simulink model "LaunchSim"  (R2022a)
settings: Solver=VariableStepAuto  StartTime=0.0  StopTime=inf  RelTol=1e-3
values from neighbouring files (symbols this model uses):
  EMFCoefCim = 18.803/1000    (= 0.018803)    [Climbing.m]    (also in Launch.m; Launching.m)
  InputLaunch = 1    [Launch.m]
  loadInertiaLaunch = 6.12 / (2*12.75) + (1.27*0.6*(0.0254^2))/2    (= 0.24024580596)    [Launch.m]
  mechDampingConstantLaunch = (TorqueCoefCim * EMFCoefCim) / TerminalResistanceCim    (= 0.000117850936333)    [Launch.m]
  ResistorTF = 12/(2*pi*1)    (= 1.9098593171)    [Launch.m]    (also in Launching.m = 0.795774715459)
  TerminalInductanceCim = 122/1000000    (= 0.000122)    [Climbing.m]    (also in Launch.m; Launching.m)
  TerminalResistanceCim = 3    [Climbing.m]    (also in Launch.m; Launching.m)
  TorqueCoefCim = 18.803/1000    (= 0.018803)    [Climbing.m]    (also in Launch.m; Launching.m)
  TorqueDisturbanceLaunch = 0    [Launch.m]
libraries: simulink_extras x3, slpidlib x1
settings Model: PacingRate=0.790000  Creator=JD Herlehy  LastModifiedBy=JD Herlehy

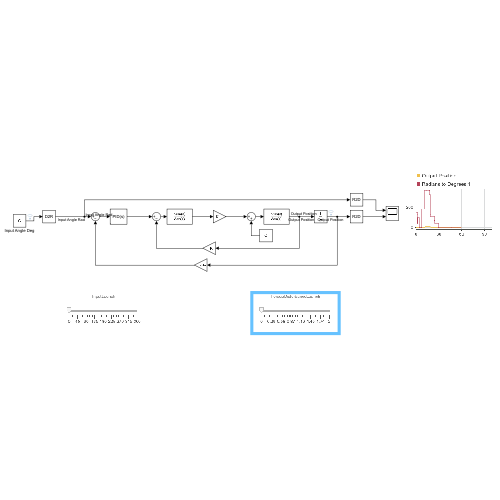
[thumbnail: Simulink's stored preview of the top-level diagram]
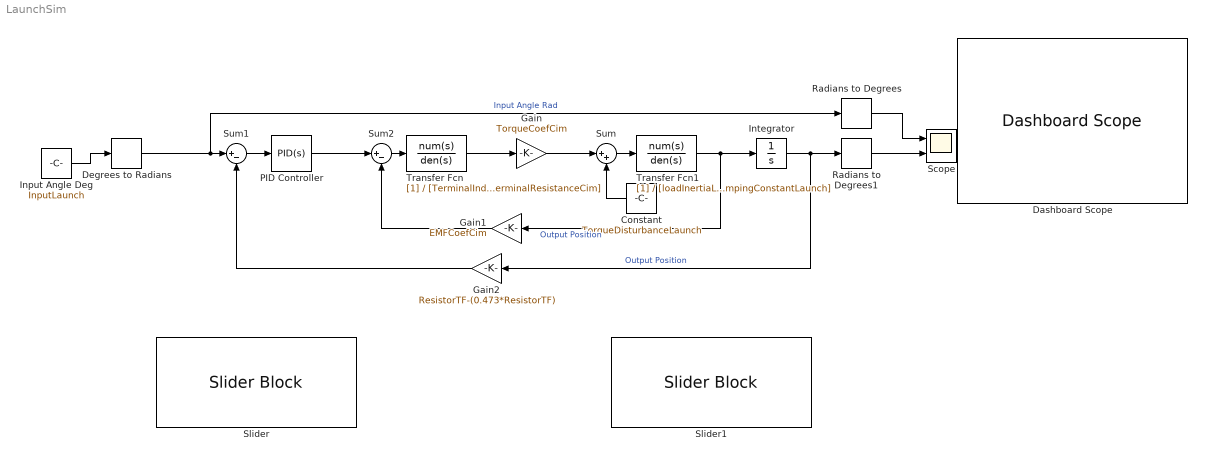
== system LaunchSim ==
  Constant : Constant  Value=TorqueDisturbanceLaunch
  Dashboard Scope : DashboardScope  Ymin=-5  Ymax=420
  Degrees to Radians : simulink_extras/Transformations/Degrees to Radians
  Gain : Gain  Gain=TorqueCoefCim
  Gain1 : Gain  Gain=EMFCoefCim
  Gain2 : Gain  Gain=ResistorTF-(0.473*ResistorTF)
  Input Angle Deg : Constant  Value=InputLaunch
  Integrator : Integrator
  PID Controller : slpidlib/PID Controller  Controller=PID  Form=Parallel  TimeDomain=Continuous-time  UseExternalTs=off  SampleTime=-1  IntegratorMethod=Forward Euler  FilterMethod=Forward Euler  ControllerParametersSource=internal  P=2.03993218165594  I=0.0170011704187148  UseKiTs=off  D=54.3843083130647  N=163.261139434515  UseFilter=on  TunerSelectOption=Transfer Function Based (PID Tuner App)  InitialConditionSource=internal  InitialConditionForIntegrator=0  InitialConditionForFilter=0  DifferentiatorICPrevScaledInput=0  ExternalReset=none  TrackingMode=off  Kt=1  LimitOutput=off  SatLimitsSource=internal  UpperSaturationLimit=inf  LowerSaturationLimit=-inf  LinearizeAsGain=on  AntiWindupMode=none  Kb=1  POutMin=[]  POutMax=[]  IOutMin=[]  IOutMax=[]  DOutMin=[]  DOutMax=[]  NOutMin=[]  NOutMax=[]  SumOutMin=[]  SumOutMax=[]  SaturationOutMin=[]  SaturationOutMax=[]  PParamMin=[]  PParamMax=[]  IParamMin=[]  IParamMax=[]  DParamMin=[]  DParamMax=[]  NParamMin=[]  NParamMax=[]  KbParamMin=[]  KbParamMax=[]  KtParamMin=[]  KtParamMax=[]  KbOutMin=[]  KbOutMax=[]  KtOutMin=[]  KtOutMax=[]  IntegratorOutMin=[]  IntegratorOutMax=[]  FilterOutMin=[]  FilterOutMax=[]  SumI1OutMin=[]  SumI1OutMax=[]  SumI2OutMin=[]  SumI2OutMax=[]  SumI3OutMin=[]  SumI3OutMax=[]  SumI4OutMin=[]  SumI4OutMax=[]  SumDOutMin=[]  SumDOutMax=[]  DifferentiatorOutMin=[]  DifferentiatorOutMax=[]  FilterDiffOutCoefMin=[]  FilterDiffOutCoefMax=[]  ReciprocalOutMin=[]  ReciprocalOutMax=[]  SumDenOutMin=[]  SumDenOutMax=[]  SumNumOutMin=[]  SumNumOutMax=[]  DivideOutMin=[]  DivideOutMax=[]  UdiffTsProdOutMin=[]  UdiffTsProdOutMax=[]  NTsProdOutMin=[]  NTsProdOutMax=[]  UintegralTsProdOutMin=[]  UintegralTsProdOutMax=[]  UngainTsProdOutMin=[]  UngainTsProdOutMax=[]  IntegratorContinuousStateAttributes=''  IntegratorStateMustResolveToSignalObject=off  IntegratorRTWStateStorageClass=Auto  FilterContinuousStateAttributes=''  FilterStateMustResolveToSignalObject=off  FilterRTWStateStorageClass=Auto  ParallelPVariant=InternalParameters  IdealPVariant=Disabled  IVariant=InternalParameters  DVariant=InternalParameters  IntegratorVariant=Continuous  SatVariant=Disabled  AWVariant=Passthrough  PCopyVariant=Disabled  TRVariant=Disabled  FdbkBlocksVariant=Forward  IdealPFdbkVariant=Disabled  SatFdbkVariant=Disabled  DerivativeFilterVariant=ContFilter  NVariant=InternalParameters  NCopyVariant=Disabled  FilterICVariant=InternalICsFilter  IntegratorICVariant=InternalICs  ExternalResetVariant=Disabled  TRSumVariant=Passthrough  SumFdbkVariant=Disabled  SumVariant=Sum_PID  TsampFilterVariant=InternalTs  TsampNgainVariant=Passthrough  TsampIntegralVariant=Passthrough  ExternalSaturationOutDataTypeStr=Inherit: Same as second input  aMode=0
  Radians to Degrees : simulink_extras/Transformations/Radians to Degrees
  Radians to Degrees1 : simulink_extras/Transformations/Radians to Degrees
  Scope : Scope  NumInputPorts=2
  Slider : SliderBlock  ScaleMax=360
  Slider1 : SliderBlock  ScaleMax=2
  Sum : Sum  Inputs=|++
  Sum1 : Sum  Inputs=|+-
  Sum2 : Sum  Inputs=|+-
  Transfer Fcn : TransferFcn  Denominator=[TerminalInductanceCim TerminalResistanceCim]
  Transfer Fcn1 : TransferFcn  Denominator=[loadInertiaLaunch mechDampingConstantLaunch]
  wires:
  Transfer Fcn/1 -> Gain/1
  Gain/1 -> Sum/1
  Sum/1 -> Transfer Fcn1/1
  Input Angle Deg/1 -> Degrees to Radians/1
  Constant/1 -> Sum/2
  Gain1/1 -> Sum2/2
  Sum2/1 -> Transfer Fcn/1
  Gain2/1 -> Sum1/2
  Degrees to Radians/1 -> Sum1/1, Radians to Degrees/1  "Input Angle Rad"
  Radians to Degrees/1 -> Scope/1
  Radians to Degrees1/1 -> Scope/2
  Sum1/1 -> PID Controller/1
  PID Controller/1 -> Sum2/1
  Transfer Fcn1/1 -> Integrator/1, Gain1/1  "Output Position"
  Integrator/1 -> Radians to Degrees1/1, Gain2/1  "Output Position"
